simulink model "s2016"  (R2018a)
settings: Solver=VariableStepAuto  StartTime=0.0  StopTime=inf  RelTol=1e-3
undefined symbols (not defined in the file or in its folder): serial
libraries: instrumentlib x3
settings Model: Creator=tomej  LastModifiedBy=tomej
settings OptimizationCC: LifeSpan=inf
settings DebuggingCC: SFExecutionAtInitializationDiag=none
settings CodeAppCC: StateflowObjectComments=on

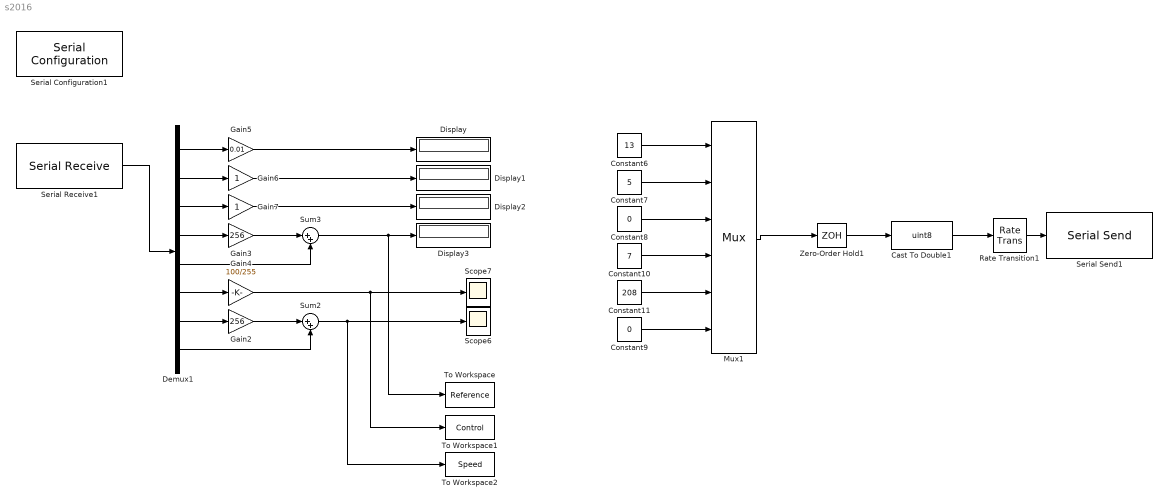
== system s2016 ==
  Cast To Double1 : DataTypeConversion  OutDataTypeStr=uint8
  Constant10 : Constant  Value=7
  Constant11 : Constant  Value=208
  Constant6 : Constant  Value=13
  Constant7 : Constant  Value=5
  Constant8 : Constant  Value=0
  Constant9 : Constant  Value=0
  Demux1 : Demux  Outputs=8
  Display{,1..3} (4 alike) : Display
  Gain2 : Gain  Gain=256
  Gain3 : Gain  Gain=256
  Gain4 : Gain  Gain=100/255
  Gain5 : Gain  Gain=0.01
  Gain6 : Gain
  Gain7 : Gain
  Mux1 : Mux  Inputs=6
      settings: DisplayOption=signals
  Rate Transition1 : RateTransition  OutPortSampleTimeOpt=Multiple of input port sample time
  Scope6 : Scope
  Scope7 : Scope
  Serial Configuration1 : instrumentlib/Serial Configuration  Priority=-200000  ComPortMenu=COM5  ComPort=COM5  ObjConstructor=serial('COM5');  BaudRate=115200  DataBits=8  Parity=none  StopBits=1  FlowControl=none  Timeout=10  ByteOrder=LittleEndian
  Serial Receive1 : instrumentlib/Serial Receive  ComPortMenu=COM5  ComPort=COM5  ObjConstructor=serial('COM5');  Header=efgh  Terminator=<none>  DataSize="[8  1]"  DataType=uint8  EnableBlockingMode=on  ActionDataUnavailable=Output last received value  CustomValue=0  SampleTime=-1
  Serial Send1 : instrumentlib/Serial Send  ComPortMenu=COM5  ComPort=COM5  ObjConstructor=serial('COM5');  Header=abcd  Terminator=<none>  EnableBlockingMode=on
  Sum2 : Sum  Inputs=|++  OutDataTypeStr=uint16
  Sum3 : Sum  Inputs=|++  OutDataTypeStr=uint16
  To Workspace : ToWorkspace  VariableName=Reference  SampleTime=-1
  To Workspace1 : ToWorkspace  VariableName=Control  SampleTime=-1
  To Workspace2 : ToWorkspace  VariableName=Speed  SampleTime=-1
  Zero-Order Hold1 : ZeroOrderHold  SampleTime=0.1
  wires:
  Serial Receive1/1 -> Demux1/1
  Gain2/1 -> Sum2/1
  Gain4/1 -> To Workspace1/1, Scope7/1
  Sum2/1 -> To Workspace2/1, Scope6/1
  Gain3/1 -> Sum3/1
  Demux1/4 -> Gain3/1
  Demux1/5 -> Sum3/2
  Demux1/6 -> Gain4/1
  Demux1/7 -> Gain2/1
  Demux1/8 -> Sum2/2
  Demux1/1 -> Gain5/1
  Gain5/1 -> Display/1
  Gain6/1 -> Display1/1
  Gain7/1 -> Display2/1
  Demux1/2 -> Gain6/1
  Demux1/3 -> Gain7/1
  Rate Transition1/1 -> Serial Send1/1
  Zero-Order Hold1/1 -> Cast To Double1/1
  Cast To Double1/1 -> Rate Transition1/1
  Constant6/1 -> Mux1/1
  Constant7/1 -> Mux1/2
  Constant8/1 -> Mux1/3
  Mux1/1 -> Zero-Order Hold1/1
  Constant9/1 -> Mux1/6
  Constant11/1 -> Mux1/5
  Constant10/1 -> Mux1/4
  Sum3/1 -> To Workspace/1, Display3/1
